simulink model "sampleModel1994"  (R2023a)
settings: Solver=VariableStepAuto  StartTime=0.0  StopTime=10.0  RelTol=1e-3
libraries: hdlsllib x2, simulink x2
settings Model: Creator=user1  LastModifiedBy=user1

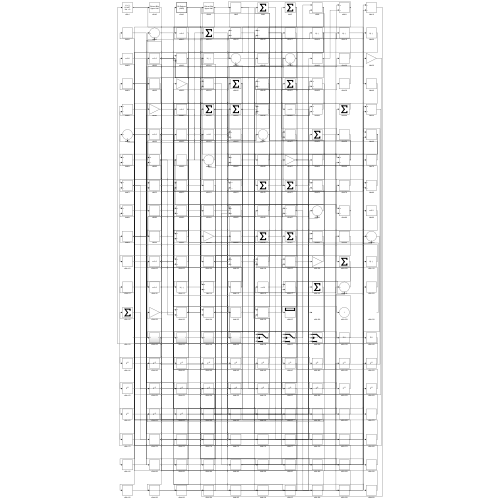
[thumbnail: Simulink's stored preview of the top-level diagram]
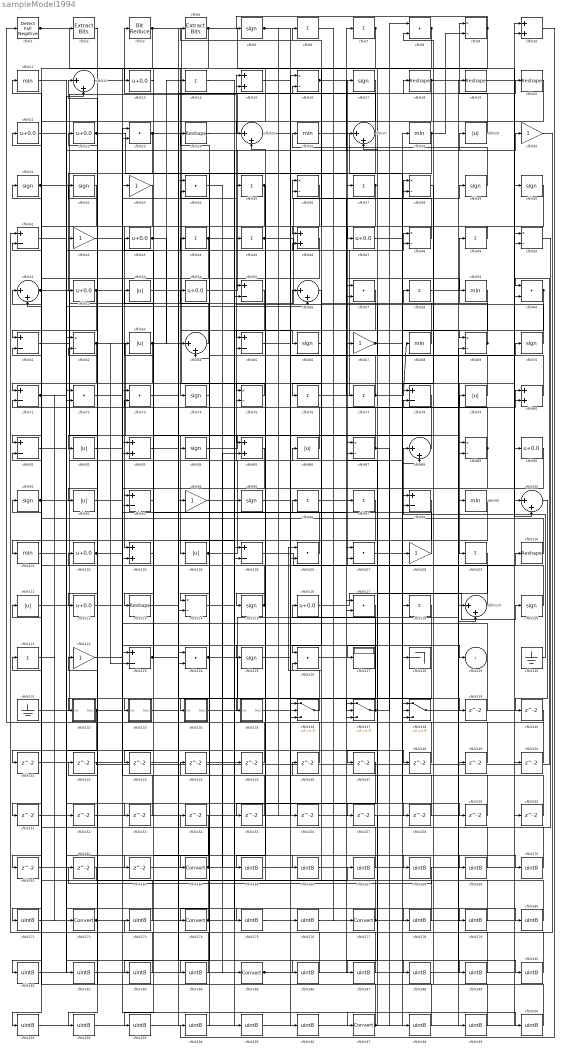
== system sampleModel1994 ==
  cfblk1 : hdlsllib/Logic and Bit Operations/Detect Fall Negative  vinit=0  OutDataTypeStr=boolean
  cfblk{10,15,46,80,83,85,103} (7 alike) : Sum
  cfblk{12,25,27,51,56,64,88,100,119} (9 alike) : Sum  Inputs=|++
  cfblk{11,26,28,59,68,99,101} (7 alike) : MinMax
  cfblk{13,21..22,43,47,52,54,90,102,112,116} (11 alike) : Bias  Bias=0.0  SaturateOnIntegerOverflow=off
  cfblk{29,53,63,79,82,86,92,104,111} (9 alike) : Abs  SaturateOnIntegerOverflow=off
  cfblk{41,55,61,65,71,78,81,93,98,105,123} (11 alike) : Sum  Inputs=+-
  cfblk{8,23,34,57,60,72..73,106..107,117,124,126} (12 alike) : DotProduct  OutDataTypeStr=Inherit: Inherit via internal rule
  cfblk{30,33,42,67,94,108,122} (7 alike) : Gain
  cfblk{6..7,14,35,37,44..45,49,58,76..77,96..97,109,118,121} (16 alike) : Sum  Inputs=+
  cfblk{18..20,24,110,113} (6 alike) : Reshape
  cfblk{9,16,36,38,48,50,62,69,75,87,89,114} (12 alike) : Product  Inputs=*/  RndMeth=Zero  SaturateOnIntegerOverflow=on
  cfblk{5,17,31..32,39..40,66,70,74,84,91,95,115,120,125} (15 alike) : Signum
  cfblk127 : Display
  cfblk128 : Terminator
  cfblk130 : Ground
  cfblk131 : Ground
  cfblk132 : Subsystem
      settings: LibrarySourceBlock=|
      | hdlsllib/Ports &
      | Subsystems/Subsystem
  cfblk133 : Subsystem
      settings: LibrarySourceBlock=|
      | hdlsllib/Ports &
      | Subsystems/Subsystem
  cfblk134 : Subsystem
      settings: LibrarySourceBlock=|
      | hdlsllib/Ports &
      | Subsystems/Subsystem
  cfblk135 : Subsystem
      settings: LibrarySourceBlock=|
      | hdlsllib/Ports &
      | Subsystems/Subsystem
  cfblk136 : Switch  SaturateOnIntegerOverflow=off  InputSameDT=off
  cfblk137 : Switch  SaturateOnIntegerOverflow=off  InputSameDT=off
  cfblk138 : Switch  SaturateOnIntegerOverflow=off  InputSameDT=off
  cfblk{139..163} (25 alike) : Delay  SampleTime=1
  cfblk{164,172,174,177,185,197} (6 alike) : DataTypeConversion  SaturateOnIntegerOverflow=off  RndMeth=Floor
  cfblk{165..171,173,175..176,178..184,186..196,198..200} (31 alike) : DataTypeConversion  OutDataTypeStr=uint8  SaturateOnIntegerOverflow=off  RndMeth=Floor
  cfblk2 : simulink/Logic and Bit Operations/Extract Bits  bitsToExtract=Upper half  numBits=8  bitIdxRange=[0 7]  outScalingMode=Preserve fixed-point scaling
      settings: LibrarySourceBlock=|
      | hdlsllib/Logic and Bit
      | Operations/Extract Bits
  cfblk3 : hdlsllib/Logic and Bit Operations/Bit Reduce  mode=AND
  cfblk4 : simulink/Logic and Bit Operations/Extract Bits  bitsToExtract=Upper half  numBits=8  bitIdxRange=[0 7]  outScalingMode=Preserve fixed-point scaling
      settings: LibrarySourceBlock=|
      | hdlsllib/Logic and Bit
      | Operations/Extract Bits
  cfblk129 : Outport  VectorParamsAs1DForOutWhenUnconnected=off
  wires:
  cfblk23/1 -> cfblk66/1, cfblk132/1(In1)
  cfblk24/1 -> cfblk20/1
  cfblk48/1 -> cfblk17/1
  cfblk33/1 -> cfblk103/1
  cfblk137/1 -> cfblk116/1, cfblk8/1
  cfblk119/1 -> cfblk37/1
  cfblk39/1 -> cfblk26/1
  cfblk71/1 -> cfblk152/1, cfblk153/1
  cfblk91/1 -> cfblk15/1, cfblk56/2, cfblk44/1
  cfblk116/1 -> cfblk120/1
  cfblk130/1 -> cfblk88/1
  cfblk2/1 -> cfblk82/1
  cfblk6/1 -> cfblk177/1
  cfblk76/1 -> cfblk48/1
  cfblk7/1 -> cfblk46/1, cfblk193/1
  cfblk66/1 -> cfblk16/2
  cfblk77/1 -> cfblk68/1, cfblk24/1
  cfblk34/1 -> cfblk185/1
  cfblk136/1 -> cfblk106/1
  cfblk105/1 -> cfblk110/1
  cfblk18/1 -> cfblk127/1, cfblk80/2, cfblk27/2, cfblk191/1
  cfblk117/1 -> cfblk164/1
  cfblk19/1 -> cfblk40/1
  cfblk51/1 -> cfblk104/1, cfblk163/1
  cfblk104/1 -> cfblk87/1, cfblk86/1
  cfblk1/1 -> cfblk74/1, cfblk2/1
  cfblk111/1 -> cfblk15/2
  cfblk62/1 -> cfblk128/1, cfblk123/2, cfblk161/1
  cfblk15/1 -> cfblk136/1
  cfblk20/1 -> cfblk133/1(In1)
  cfblk27/1 -> cfblk3/1, cfblk64/2
  cfblk92/1 -> cfblk33/1
  cfblk32/1 -> cfblk52/1
  cfblk88/1 -> cfblk84/1
  cfblk56/1 -> cfblk76/1
  cfblk93/1 -> cfblk43/1
  cfblk138/1 -> cfblk100/1
  cfblk8/1 -> cfblk25/1, cfblk61/1
  cfblk106/1 -> cfblk25/2
  cfblk79/1 -> cfblk57/1
  cfblk45/1 -> cfblk48/2, cfblk135/1(In1)
  cfblk54/1 -> cfblk7/1
  cfblk86/1 -> cfblk22/1
  cfblk22/1 -> cfblk57/2, cfblk55/2, cfblk114/2
  cfblk132/1(Out1) -> cfblk171/1, cfblk200/1
  cfblk31/1 -> cfblk29/1, cfblk158/1
  cfblk37/1 -> cfblk83/2, cfblk36/2
  cfblk67/1 -> cfblk69/1, cfblk139/1
  cfblk61/1 -> cfblk39/1
  cfblk90/1 -> cfblk106/2
  cfblk98/1 -> cfblk174/1
  cfblk16/1 -> cfblk77/1, cfblk59/1
  cfblk43/1 -> cfblk113/1, cfblk64/1
  cfblk53/1 -> cfblk109/1
  cfblk38/1 -> cfblk78/1
  cfblk68/1 -> cfblk36/1
  cfblk112/1 -> cfblk97/1
  cfblk97/1 -> cfblk101/1
  cfblk80/1 -> cfblk45/1
  cfblk64/1 -> cfblk54/1
  cfblk28/1 -> cfblk42/1, cfblk9/2
  cfblk60/1 -> cfblk126/1, cfblk85/1
  cfblk123/1 -> cfblk73/2, cfblk18/1, cfblk46/2
  cfblk49/1 -> cfblk47/1
  cfblk26/1 -> cfblk88/2
  cfblk89/1 -> cfblk115/1, cfblk75/2
  cfblk115/1 -> cfblk32/1, cfblk81/2
  cfblk125/1 -> cfblk70/1
  cfblk82/1 -> cfblk35/1
  cfblk131/1 -> cfblk80/1
  cfblk63/1 -> cfblk112/1, cfblk14/1
  cfblk75/1 -> cfblk71/1
  cfblk29/1 -> cfblk9/1
  cfblk78/1 -> cfblk93/1
  cfblk25/1 -> cfblk19/1
  cfblk52/1 -> cfblk125/1, cfblk151/1, cfblk166/1
  cfblk84/1 -> cfblk89/1
  cfblk122/1 -> cfblk197/1
  cfblk4/1 -> cfblk100/2, cfblk23/2
  cfblk83/1 -> cfblk105/2
  cfblk96/1 -> cfblk79/1
  cfblk103/1 -> cfblk63/1
  cfblk107/1 -> cfblk28/1
  cfblk85/1 -> cfblk103/2
  cfblk35/1 -> cfblk92/1, cfblk75/1
  cfblk102/1 -> cfblk56/1, cfblk129/1
  cfblk3/1 -> cfblk136/2, cfblk13/1, cfblk138/2
  cfblk120/1 -> cfblk102/1
  cfblk126/1 -> cfblk38/1
  cfblk124/1 -> cfblk137/2, cfblk30/1
  cfblk81/1 -> cfblk27/1
  cfblk5/1 -> cfblk89/2, cfblk156/1
  cfblk44/1 -> cfblk81/1, cfblk145/1, cfblk170/1
  cfblk9/1 -> cfblk5/1, cfblk157/1
  cfblk69/1 -> cfblk4/1, cfblk49/1
  cfblk70/1 -> cfblk55/1
  cfblk121/1 -> cfblk172/1
  cfblk87/1 -> cfblk71/2, cfblk198/1
  cfblk134/1(Out1) -> cfblk99/1
  cfblk108/1 -> cfblk53/1
  cfblk55/1 -> cfblk65/1
  cfblk36/1 -> cfblk124/2
  cfblk74/1 -> cfblk134/1(In1)
  cfblk46/1 -> cfblk114/1
  cfblk110/1 -> cfblk51/1
  cfblk57/1 -> cfblk136/3
  cfblk133/1(Out1) -> cfblk96/1
  cfblk139/1 -> cfblk73/1
  cfblk100/1 -> cfblk140/1
  cfblk140/1 -> cfblk1/1
  cfblk17/1 -> cfblk141/1
  cfblk141/1 -> cfblk93/2
  cfblk142/1 -> cfblk60/1
  cfblk13/1 -> cfblk143/1
  cfblk143/1 -> cfblk124/1
  cfblk144/1 -> cfblk105/1
  cfblk145/1 -> cfblk51/2
  cfblk146/1 -> cfblk62/1
  cfblk109/1 -> cfblk147/1
  cfblk101/1 -> cfblk148/1
  cfblk148/1 -> cfblk126/2
  cfblk149/1 -> cfblk61/2
  cfblk150/1 -> cfblk8/2
  cfblk151/1 -> cfblk137/3
  cfblk152/1 -> cfblk16/1
  cfblk153/1 -> cfblk23/1
  cfblk50/1 -> cfblk154/1
  cfblk59/1 -> cfblk155/1
  cfblk155/1 -> cfblk83/1
  cfblk156/1 -> cfblk69/2
  cfblk158/1 -> cfblk87/2
  cfblk47/1 -> cfblk159/1
  cfblk159/1 -> cfblk123/1
  cfblk160/1 -> cfblk78/2
  cfblk161/1 -> cfblk119/2
  cfblk163/1 -> cfblk38/2
  cfblk164/1 -> cfblk150/1, cfblk138/3, cfblk85/2, cfblk21/1
  cfblk147/1 -> cfblk165/1
  cfblk165/1 -> cfblk117/1
  cfblk166/1 -> cfblk117/2
  cfblk162/1 -> cfblk167/1
  cfblk167/1 -> cfblk107/1
  cfblk42/1 -> cfblk168/1
  cfblk168/1 -> cfblk162/1
  cfblk72/1 -> cfblk169/1
  cfblk169/1 -> cfblk146/1
  cfblk170/1 -> cfblk72/1
  cfblk171/1 -> cfblk72/2
  cfblk172/1 -> cfblk90/1, cfblk50/2, cfblk95/1
  cfblk30/1 -> cfblk173/1
  cfblk173/1 -> cfblk121/1
  cfblk174/1 -> cfblk108/1, cfblk91/1
  cfblk21/1 -> cfblk175/1
  cfblk175/1 -> cfblk98/1
  cfblk95/1 -> cfblk176/1
  cfblk176/1 -> cfblk98/2
  cfblk177/1 -> cfblk149/1, cfblk65/2, cfblk111/1
  cfblk14/1 -> cfblk178/1
  cfblk178/1 -> cfblk6/1
  cfblk12/1 -> cfblk179/1
  cfblk179/1 -> cfblk142/1
  cfblk135/1(Out1) -> cfblk180/1
  cfblk180/1 -> cfblk12/1
  cfblk40/1 -> cfblk181/1
  cfblk181/1 -> cfblk12/2
  cfblk41/1 -> cfblk182/1
  cfblk182/1 -> cfblk60/2
  cfblk154/1 -> cfblk183/1
  cfblk183/1 -> cfblk41/1
  cfblk99/1 -> cfblk184/1
  cfblk184/1 -> cfblk41/2
  cfblk185/1 -> cfblk160/1, cfblk50/1, cfblk67/1
  cfblk73/1 -> cfblk186/1
  cfblk186/1 -> cfblk34/1
  cfblk157/1 -> cfblk187/1
  cfblk187/1 -> cfblk34/2
  cfblk11/1 -> cfblk188/1
  cfblk188/1 -> cfblk119/1
  cfblk113/1 -> cfblk189/1
  cfblk189/1 -> cfblk11/1
  cfblk94/1 -> cfblk190/1
  cfblk190/1 -> cfblk137/1
  cfblk191/1 -> cfblk94/1
  cfblk118/1 -> cfblk192/1
  cfblk192/1 -> cfblk138/1
  cfblk193/1 -> cfblk118/1
  cfblk10/1 -> cfblk194/1
  cfblk194/1 -> cfblk144/1
  cfblk114/1 -> cfblk195/1
  cfblk195/1 -> cfblk10/1
  cfblk65/1 -> cfblk196/1
  cfblk196/1 -> cfblk10/2
  cfblk197/1 -> cfblk107/2, cfblk62/2
  cfblk198/1 -> cfblk122/1
  cfblk58/1 -> cfblk199/1
  cfblk199/1 -> cfblk31/1
  cfblk200/1 -> cfblk58/1

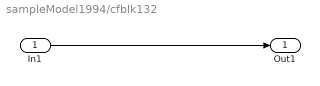
== system sampleModel1994/cfblk132 ==
  In1 : Inport
  Out1 : Outport
  wires:
  In1/1 -> Out1/1

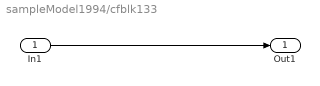
== system sampleModel1994/cfblk133 ==
  In1 : Inport
  Out1 : Outport
  wires:
  In1/1 -> Out1/1

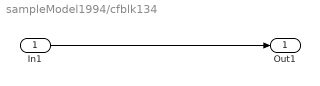
== system sampleModel1994/cfblk134 ==
  In1 : Inport
  Out1 : Outport
  wires:
  In1/1 -> Out1/1

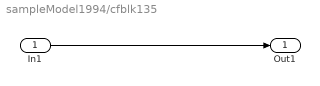
== system sampleModel1994/cfblk135 ==
  In1 : Inport
  Out1 : Outport
  wires:
  In1/1 -> Out1/1
